simulink model "Bloque"  (R2026a)
settings: Solver=ode15s  MaxStep=1e-6
values from neighbouring files (symbols this model uses):
  Pp = 3    [coeficientes.m]
libraries: eeTransforms x1
settings Model: Creator=admin  LastModifiedBy=admin
settings SolverCC: SolverResetMethod=Robust

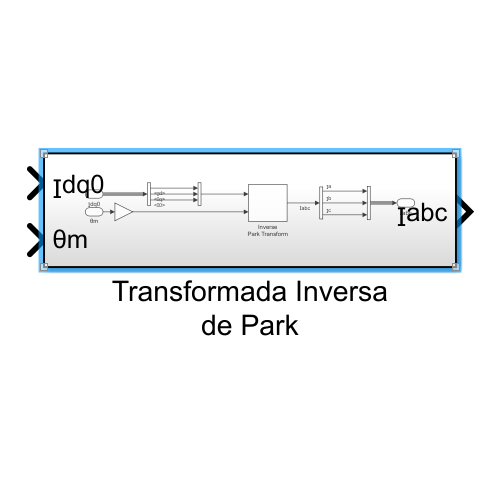
[thumbnail: Simulink's stored preview of the top-level diagram]
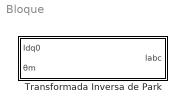
== system Bloque ==
  Transformada Inversa de Park : Subsystem

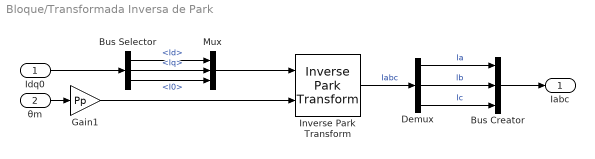
== system Bloque/Transformada Inversa de Park ==
  Ⅰdq0 : Inport
  θm : Inport  Port=2
  Bus Creator : BusCreator  Inputs=3
  Bus Selector : BusSelector  OutputSignals=Ⅰd,Ⅰq,Ⅰ0
  Demux : Demux  Outputs=3
  Gain1 : Gain  Gain=Pp
  Inverse Park Transform : eeTransforms/Inverse Park Transform  AxisAlignment=Q-axis  PowerInvariant=off
      settings: LibrarySourceBlock=|
      | ee_sl_lib/Mathematical
      | Transforms/Inverse
      | Park Transform
  Mux : Mux  Inputs=3
  Ⅰabc : Outport
  wires:
  Gain1/1 -> Inverse Park Transform/2
  Ⅰdq0/1 -> Bus Selector/1
  θm/1 -> Gain1/1
  Demux/1 -> Bus Creator/1  "Ⅰa"
  Inverse Park Transform/1 -> Demux/1  "Ⅰabc"
  Demux/2 -> Bus Creator/2  "Ⅰb"
  Bus Creator/1 -> Ⅰabc/1
  Demux/3 -> Bus Creator/3  "Ⅰc"
  Bus Selector/1 -> Mux/1  "<Ⅰd>"
  Bus Selector/2 -> Mux/2  "<Ⅰq>"
  Bus Selector/3 -> Mux/3  "<Ⅰ0>"
  Mux/1 -> Inverse Park Transform/1
